simulink model "Q4_W2"  (R2020b)
settings: Solver=VariableStepAuto  StartTime=0.0  StopTime=10.0  RelTol=1e-3
settings Model: Creator=hp  LastModifiedBy=hp

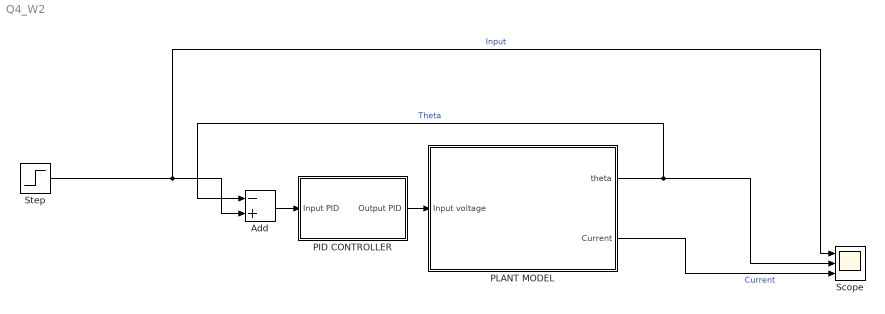
== system Q4_W2 ==
  Add : Sum  Inputs=-+
  PID CONTROLLER : Subsystem
  PLANT MODEL : Subsystem
  Scope : Scope  NumInputPorts=3
  Step : Step  SampleTime=0
  wires:
  PLANT MODEL/1(theta) -> Add/1, Scope/2  "Theta"
  PLANT MODEL/2(Current) -> Scope/3  "Current"
  Step/1 -> Add/2, Scope/1  "Input"
  PID CONTROLLER/1(Output PID) -> PLANT MODEL/1(Input voltage)
  Add/1 -> PID CONTROLLER/1(Input PID)

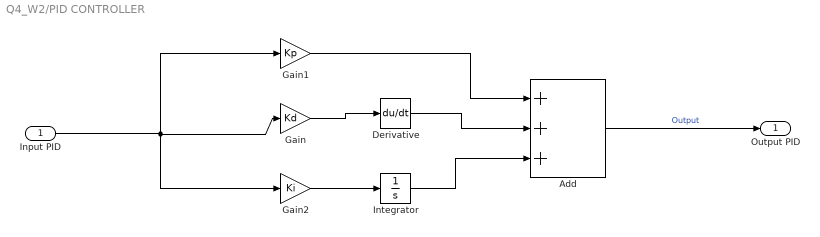
== system Q4_W2/PID CONTROLLER ==
  Input PID : Inport
  Add : Sum  Inputs=+++
  Derivative : Derivative
  Gain : Gain  Gain=Kd  mask{Kd=23}
  Gain1 : Gain  Gain=Kp  mask{Kp=612}
  Gain2 : Gain  Gain=Ki  mask{Ki=0.17028}
  Integrator : Integrator
  Output PID : Outport
  wires:
  Gain1/1 -> Add/1
  Gain2/1 -> Integrator/1
  Add/1 -> Output PID/1  "Output"
  Input PID/1 -> Gain/1, Gain2/1, Gain1/1
  Integrator/1 -> Add/3
  Gain/1 -> Derivative/1
  Derivative/1 -> Add/2

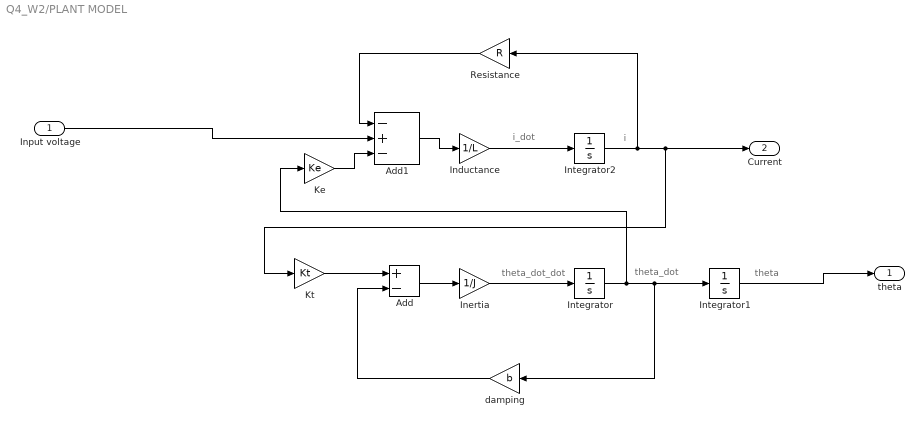
== system Q4_W2/PLANT MODEL ==
  note: i_dot
  note: theta_dot_dot
  note: i
  note: theta
  note: theta_dot
  Input voltage : Inport
  Add : Sum  Inputs=+-
  Add1 : Sum  Inputs=-+-
  Inductance : Gain  Gain=1/L  mask{L=2.75E-6}
  Inertia : Gain  Gain=1/J  mask{J=3.2284E-6}
  Integrator : Integrator
  Integrator1 : Integrator
  Integrator2 : Integrator
  Ke : Gain  Gain=Ke  mask{Ke=0.0274}
  Kt : Gain  Gain=Kt  mask{Kt=0.0274}
  Resistance : Gain  Gain=R  mask{R=4}
  damping : Gain  Gain=b  mask{b=3.5077E-6}
  theta : Outport
  Current : Outport  Port=2
  wires:
  Integrator/1 -> Ke/1, damping/1, Integrator1/1
  Inductance/1 -> Integrator2/1
  Add/1 -> Inertia/1
  Kt/1 -> Add/1
  Add1/1 -> Inductance/1
  damping/1 -> Add/2
  Inertia/1 -> Integrator/1
  Ke/1 -> Add1/3
  Resistance/1 -> Add1/1
  Integrator2/1 -> Resistance/1, Current/1, Kt/1
  Input voltage/1 -> Add1/2
  Integrator1/1 -> theta/1
